simulink model "AS_PatientInterface_VerifierModel"  (R2022b)
settings: Solver=VariableStepAuto  StartTime=0.0  StopTime=30.0  RelTol=1e-3
model workspace (MAT data in the model file):
  T_humidifier = 40
undefined symbols (not defined in the file): D_tube
libraries: fl_lib x17, nesl_utility x3
settings Model: DataDictionary=AS_DataDictionary.sldd  Creator=CSN-Simulation  LastModifiedBy=MATLAB
settings DebuggingCC: UnconnectedInputMsg=warning  UnconnectedOutputMsg=warning  UnconnectedLineMsg=warning
settings ModelReferenceCC: EnableRefExpFcnMdlSchedulingChecks=on
settings RTWCC: DLArmComputeVersion=19.05

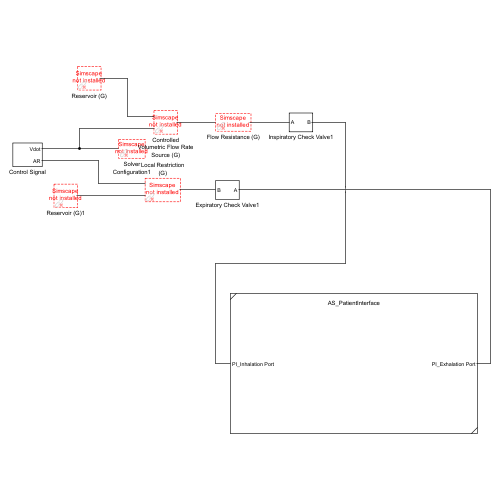
[thumbnail: Simulink's stored preview of the top-level diagram]
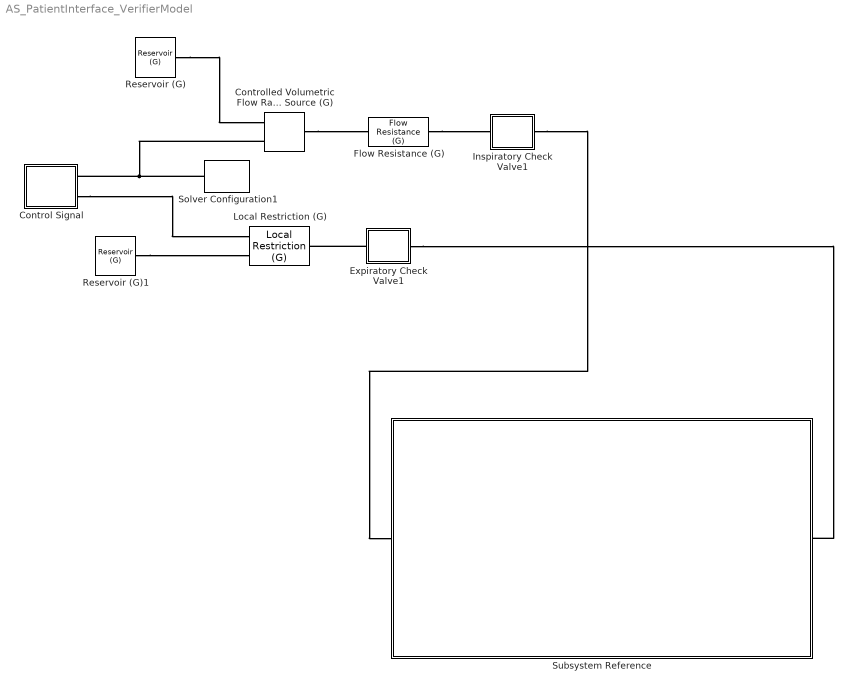
== system AS_PatientInterface_VerifierModel ==
  Control Signal : Subsystem  Tag=PublishSubsystem  mask(Control Signal){tidal_volume=0.5, respiratory_rate=15, IE_ratio=1/3}
      mask prompts: tidal_volume "Tidal Volume (L)"; respiratory_rate "Respiratory Rate (breaths/min)"; IE_ratio "Inspiration to Expiration Ratio"
      mask help: This subsystem generates the input signals that controls the inspiratory flow and expiratory valve.
  Controlled Volumetric Flow Rate Source (G) : fl_lib/Gas/Sources/Controlled Volumetric Flow Rate Source (G)  power_spec=foundation.enum.power_spec.isentropic  area_A=pi*D_tube^2/4 m^2  area_B=pi*D_tube^2/4 m^2
      settings: InternalSimscapePortConfiguration="{\"Bottom\":[],\"Left\":[{\"id\":\"A\",\"label\":\"A\",\"type\":\"foundation.gas.gas\"},{\"id\":\"V\",\"label\":\"V\",\"type\":\"input\"}],\"Right\":[{\"id\":\"B\",\"label\":\"B\",\"type\":\"foundation.gas.gas\"}],\"Top\":[]}"
  Expiratory Check Valve1 : Subsystem  mask(Check Valve){p_max=1e3, p_crack=10, A_max=pi*(0.9*D_tube)^2/4, A_leak=1e-10, A_port=pi*D_tube^2/4, Cd=0.8, tau=0.1}
      mask prompts: p_max "Max opening pressure differential (Pa)"; p_crack "Cracking pressure differential (Pa)"; A_max "Max opening area (m^2)"; A_leak "Leakage area (m^2)"; A_port "Connecting port area (m^2)"; Cd "Discharge coefficient"; tau "Opening time constant (s)"
      mask help: This subsystem models a check valve that permits flow from port A to port B but restricts flow from port B to port A.
  Flow Resistance (G) : fl_lib/Gas/Elements/Flow Resistance (G)  delta_p_nominal=100 Pa  mdot_nominal=0.5 g/s  rho_nominal=0 kg/m^3  area=pi*D_tube^2/4 m^2  laminar_fraction=1e-3
      settings: InternalSimscapePortConfiguration="{\"Bottom\":[],\"Left\":[{\"id\":\"A\",\"label\":\"A\",\"type\":\"foundation.gas.gas\"}],\"Right\":[{\"id\":\"B\",\"label\":\"B\",\"type\":\"foundation.gas.gas\"}],\"Top\":[]}"
  Inspiratory Check Valve1 : Subsystem  Tag=PublishSubsystem  mask(Check Valve){p_max=1e3, p_crack=10, A_max=pi*(0.9*D_tube)^2/4, A_leak=1e-10, A_port=pi*D_tube^2/4, Cd=0.8, tau=0.1}
      mask prompts: p_max "Max opening pressure differential (Pa)"; p_crack "Cracking pressure differential (Pa)"; A_max "Max opening area (m^2)"; A_leak "Leakage area (m^2)"; A_port "Connecting port area (m^2)"; Cd "Discharge coefficient"; tau "Opening time constant (s)"
      mask help: This subsystem models a check valve that permits flow from port A to port B but restricts flow from port B to port A.
  Local Restriction (G) : fl_lib/Gas/Elements/Local Restriction (G)  restriction_type=foundation.enum.restriction_type.variable  restriction_area=1e-3 m^2  min_area=1e-10 m^2  max_area=pi*(0.9*D_tube)^2/4 m^2  area=pi*D_tube^2/4 m^2  Cd=0.64  B_lam=0.999
      settings: InternalSimscapePortConfiguration="{\"Bottom\":[],\"Left\":[{\"id\":\"A\",\"label\":\"A\",\"type\":\"foundation.gas.gas\"},{\"id\":\"area_in\",\"label\":\"AR\",\"type\":\"input\"}],\"Right\":[{\"id\":\"B\",\"label\":\"B\",\"type\":\"foundation.gas.gas\"}],\"Top\":[]}"
  Reservoir (G) : fl_lib/Gas/Elements/Reservoir (G)  pressure_spec=foundation.enum.pressure_spec.atmospheric  reservoir_pressure=0.101325 MPa  reservoir_temperature=T_room degC  area_A=pi*D_tube^2/4 m^2
  Reservoir (G)1 : fl_lib/Gas/Elements/Reservoir (G)  pressure_spec=foundation.enum.pressure_spec.atmospheric  reservoir_pressure=0.101325 MPa  reservoir_temperature=T_room degC  area_A=pi*D_tube^2/4 m^2
  Solver Configuration1 : nesl_utility/Solver Configuration  PhysicalDomain=network_engine_domain  SubClassName=solver  LeftPortType=input  RightPortType=generic  Tones=[]  Harmonics=[]  SimulateNoise=off  Profile=off  UseLocalSampling=off  EnableSwitchedLinearOptims=on  FrequencyDomain=off  UseCCode=off  RelTol=0.001  AbsTol=1e-06  MinStep=1e-09  ToWorkspace=off  RevertToSquareIcSolve=off  NumHomotopyIterations=100  PhasorMode=off  PhasorModeNumHarmonics=1  DoDC=off  ResidualTolerance=1e-9  UseLocalSolver=off  LocalSolverChoice=NE_BACKWARD_EULER_ADVANCER  LocalSolverSampleTime=0.01  DoFixedCost=off  MaxNonlinIter=3  MaxModeIter=2  ComputeImpulses=off  ImpulseIterations=2  LinearAlgebra=auto  EquationFormulation=NE_TIME_EF  DelaysMemoryBudget=1024  AutomaticFiltering=on  FilteringTimeConstant=0.001  PartitionStorageMethod=AS_NEEDED  PartitionMemoryBudget=1024  PartitionMethod=FAST
  Subsystem Reference : Subsystem  ReferencedSubsystem=AS_PatientInterface
  connections:
  Solver Configuration1/RConn1 -- Controlled Volumetric Flow Rate Source (G)/LConn2 -- Control Signal/RConn1
  Reservoir (G)/LConn1 -- Controlled Volumetric Flow Rate Source (G)/LConn1
  Controlled Volumetric Flow Rate Source (G)/RConn1 -- Flow Resistance (G)/LConn1
  Reservoir (G)1/LConn1 -- Local Restriction (G)/LConn1
  Control Signal/RConn2 -- Local Restriction (G)/LConn2
  Flow Resistance (G)/RConn1 -- Inspiratory Check Valve1/LConn1
  Inspiratory Check Valve1/RConn1 -- Subsystem Reference/LConn1
  Expiratory Check Valve1/RConn1 -- Local Restriction (G)/RConn1
  Expiratory Check Valve1/LConn1 -- Subsystem Reference/RConn1

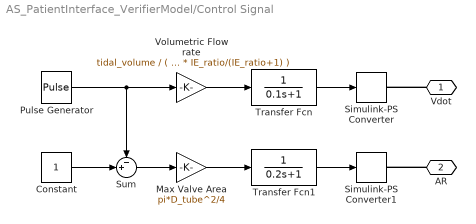
== system AS_PatientInterface_VerifierModel/Control Signal ==
  Constant : Constant
  Max Valve Area : Gain  Gain=pi*D_tube^2/4
  Pulse Generator : DiscretePulseGenerator  PulseType=Time based  Period=60 / respiratory_rate  PulseWidth=IE_ratio/(IE_ratio+1) * 100
  Simulink-PS Converter : nesl_utility/Simulink-PS Converter  PhysicalDomain=network_engine_domain  SubClassName=ps_input  LeftPortType=input  RightPortType=output  PseudoPeriodic=off  Frequencies=[]  NoiseDistribution=none  NoiseParameters=[]  Unit=l/s  AffineConversion=off  FilteringAndDerivatives=provide  SimscapeFilterOrder=1  InputFilterTimeConstant=0.001  UdotUserProvided=0
  Simulink-PS Converter1 : nesl_utility/Simulink-PS Converter  PhysicalDomain=network_engine_domain  SubClassName=ps_input  LeftPortType=input  RightPortType=output  PseudoPeriodic=off  Frequencies=[]  NoiseDistribution=none  NoiseParameters=[]  Unit=m^2  AffineConversion=off  FilteringAndDerivatives=provide  SimscapeFilterOrder=1  InputFilterTimeConstant=0.001  UdotUserProvided=0
  Sum : Sum  Inputs=-+|
  Transfer Fcn : TransferFcn  Denominator=[0.1 1]
  Transfer Fcn1 : TransferFcn  Denominator=[0.2 1]
  Volumetric Flow rate : Gain  Gain=tidal_volume / ( (60/respiratory_rate) * IE_ratio/(IE_ratio+1) )
  Vdot : PMIOPort  Side=Right
  AR : PMIOPort  Port=2  Side=Right
  wires:
  Constant/1 -> Sum/2
  Pulse Generator/1 -> Sum/1, Volumetric Flow rate/1
  Volumetric Flow rate/1 -> Transfer Fcn/1
  Max Valve Area/1 -> Transfer Fcn1/1
  Transfer Fcn/1 -> Simulink-PS Converter/1
  Transfer Fcn1/1 -> Simulink-PS Converter1/1
  Sum/1 -> Max Valve Area/1
  connections:
  Vdot/RConn1 -- Simulink-PS Converter/RConn1
  AR/RConn1 -- Simulink-PS Converter1/RConn1

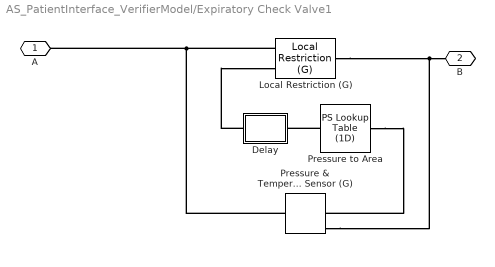
== system AS_PatientInterface_VerifierModel/Expiratory Check Valve1 ==
  Delay : Subsystem  mask{tau=tau, x0=A_leak}
      mask prompts: tau "Time constant (s)"; x0 "Initial output"
  Local Restriction (G) : fl_lib/Gas/Elements/Local Restriction (G)  restriction_type=foundation.enum.restriction_type.variable  restriction_area=1e-3 m^2  min_area=A_leak/2 m^2  max_area=(A_max + A_port)/2 m^2  area=A_port m^2  Cd=Cd  B_lam=0.999
      settings: InternalSimscapePortConfiguration="{\"Bottom\":[],\"Left\":[{\"id\":\"A\",\"label\":\"A\",\"type\":\"foundation.gas.gas\"},{\"id\":\"area_in\",\"label\":\"AR\",\"type\":\"input\"}],\"Right\":[{\"id\":\"B\",\"label\":\"B\",\"type\":\"foundation.gas.gas\"}],\"Top\":[]}"
  Pressure & Temperature Sensor (G) : fl_lib/Gas/Sensors/Pressure & Temperature Sensor (G)
      settings: InternalSimscapePortConfiguration="{\"Bottom\":[],\"Left\":[{\"id\":\"A\",\"label\":\"A\",\"type\":\"foundation.gas.gas\"}],\"Right\":[{\"id\":\"B\",\"label\":\"B\",\"type\":\"foundation.gas.gas\"},{\"id\":\"P\",\"label\":\"P\",\"type\":\"output\"},{\"id\":\"T\",\"label\":\"T\",\"type\":\"output\"}],\"Top\":[]}"
  Pressure to Area : fl_lib/Physical Signals/Lookup Tables/PS Lookup Table (1D)  x=[-0.2 -0.1 0 0.2 0.5 0.8 1 1.1 1.2]*(p_max - p_crack) + p_crack Pa  f=[0 0 0 0.2 0.5 0.8 1 1 1]*(A_max - A_leak) + A_leak m^2  interp_method=simscape.enum.interpolation.smooth  extrap_method=simscape.enum.extrapolation.linear
  A : PMIOPort  Side=Left
  B : PMIOPort  Port=2  Side=Right
  connections:
  Pressure to Area/RConn1 -- Delay/LConn1
  Local Restriction (G)/LConn1 -- Pressure & Temperature Sensor (G)/LConn1 -- A/RConn1
  Delay/RConn1 -- Local Restriction (G)/LConn2
  Pressure & Temperature Sensor (G)/RConn1 -- Local Restriction (G)/RConn1 -- B/RConn1
  Pressure to Area/LConn1 -- Pressure & Temperature Sensor (G)/RConn2

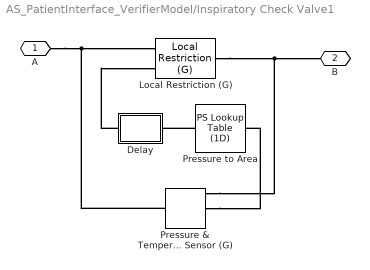
== system AS_PatientInterface_VerifierModel/Inspiratory Check Valve1 ==
  Delay : Subsystem  mask{tau=tau, x0=A_leak}
      mask prompts: tau "Time constant (s)"; x0 "Initial output"
  Local Restriction (G) : fl_lib/Gas/Elements/Local Restriction (G)  restriction_type=foundation.enum.restriction_type.variable  restriction_area=1e-3 m^2  min_area=A_leak/2 m^2  max_area=(A_max + A_port)/2 m^2  area=A_port m^2  Cd=Cd  B_lam=0.999
      settings: InternalSimscapePortConfiguration="{\"Bottom\":[],\"Left\":[{\"id\":\"A\",\"label\":\"A\",\"type\":\"foundation.gas.gas\"},{\"id\":\"area_in\",\"label\":\"AR\",\"type\":\"input\"}],\"Right\":[{\"id\":\"B\",\"label\":\"B\",\"type\":\"foundation.gas.gas\"}],\"Top\":[]}"
  Pressure & Temperature Sensor (G) : fl_lib/Gas/Sensors/Pressure & Temperature Sensor (G)
      settings: InternalSimscapePortConfiguration="{\"Bottom\":[],\"Left\":[{\"id\":\"A\",\"label\":\"A\",\"type\":\"foundation.gas.gas\"}],\"Right\":[{\"id\":\"B\",\"label\":\"B\",\"type\":\"foundation.gas.gas\"},{\"id\":\"P\",\"label\":\"P\",\"type\":\"output\"},{\"id\":\"T\",\"label\":\"T\",\"type\":\"output\"}],\"Top\":[]}"
  Pressure to Area : fl_lib/Physical Signals/Lookup Tables/PS Lookup Table (1D)  x=[-0.2 -0.1 0 0.2 0.5 0.8 1 1.1 1.2]*(p_max - p_crack) + p_crack Pa  f=[0 0 0 0.2 0.5 0.8 1 1 1]*(A_max - A_leak) + A_leak m^2  interp_method=simscape.enum.interpolation.smooth  extrap_method=simscape.enum.extrapolation.linear
  A : PMIOPort  Side=Left
  B : PMIOPort  Port=2  Side=Right
  connections:
  Pressure to Area/RConn1 -- Delay/LConn1
  Pressure & Temperature Sensor (G)/RConn2 -- Pressure to Area/LConn1
  A/RConn1 -- Pressure & Temperature Sensor (G)/LConn1 -- Local Restriction (G)/LConn1
  Local Restriction (G)/RConn1 -- Pressure & Temperature Sensor (G)/RConn1 -- B/RConn1
  Delay/RConn1 -- Local Restriction (G)/LConn2

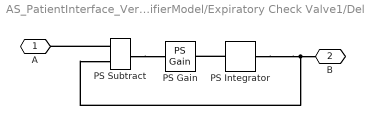
== system AS_PatientInterface_VerifierModel/Expiratory Check Valve1/Delay ==
  PS Gain : fl_lib/Physical Signals/Functions/PS Gain  gain=1/tau 1/s
  PS Integrator : fl_lib/Physical Signals/Linear Operators/PS Integrator  reset_method=foundation.enum.IntegratorResetSpec.None  initial_condition_spec=foundation.enum.IntegratorICSpec.Internal  x0=x0 m^2
  PS Subtract : fl_lib/Physical Signals/Functions/PS Subtract
  A : PMIOPort  Side=Left
  B : PMIOPort  Port=2  Side=Right
  connections:
  PS Integrator/LConn1 -- PS Gain/RConn1
  PS Subtract/LConn1 -- A/RConn1
  PS Subtract/RConn1 -- PS Gain/LConn1
  B/RConn1 -- PS Subtract/LConn2 -- PS Integrator/RConn1

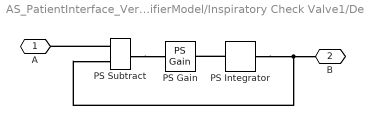
== system AS_PatientInterface_VerifierModel/Inspiratory Check Valve1/Delay ==
  PS Gain : fl_lib/Physical Signals/Functions/PS Gain  gain=1/tau 1/s
  PS Integrator : fl_lib/Physical Signals/Linear Operators/PS Integrator  reset_method=foundation.enum.IntegratorResetSpec.None  initial_condition_spec=foundation.enum.IntegratorICSpec.Internal  x0=x0 m^2
  PS Subtract : fl_lib/Physical Signals/Functions/PS Subtract
  A : PMIOPort  Side=Left
  B : PMIOPort  Port=2  Side=Right
  connections:
  PS Integrator/RConn1 -- PS Subtract/LConn2 -- B/RConn1
  PS Subtract/RConn1 -- PS Gain/LConn1
  PS Subtract/LConn1 -- A/RConn1
  PS Integrator/LConn1 -- PS Gain/RConn1
